simulink model "fzinfer_example"  (Simulink 6.2)
settings: Solver=ode45  StartTime=0.0  StopTime=4  FixedStep=.25  RelTol=1e-3
undefined symbols (not defined in the file): mfs, rls
libraries: simulink x1
settings Model: Creator=lbusoniu  LastModifiedBy=Administrator  ExtModeAutoUpdateStatusClock=off
settings DataIOCC: SignalLoggingName=sigsOut
settings HardwareCC: TargetUnknown=on

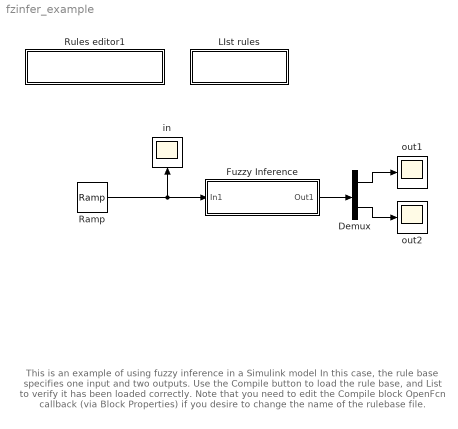
== system fzinfer_example ==
  note: This is an example of using fuzzy inference in a Simulink model
      |
      | In this case, the rule base specifies one input and two outputs.
      | Use the Compile button to load the rule base, and List to verify
      | it has been loaded correctly. Note that you need to edit the
      | Compile block OpenFcn callback (via Block Properties)
      | if you desire to change the name of the rulebase file.
  Demux : Demux  Outputs=2
  Fuzzy Inference : Subsystem  mask(Fuzzy inference block){rls=rls, mfs=mfs, def=[1 3]}
      mask prompts: rls "Rule matrix:"; mfs "Membership functions matrix:"; def "Default output:"
      mask help:
      | MIN-MAX inference with
      |  fuzzy means defuzzification
      mask Help: Fuzzy inference block can be used as a direct fuzzy controller or as a fuzzy supervisor. For details on dialog parameters see INFER.
      mask Display: disp('Fuzzy Inference')
  LIst rules : Subsystem  Orientation=down
      settings: OpenFcn=disp(rls2txt(rls, mfs, inputs, outputs, nlab, labels));
      mask Display: disp('List Fuzzy Rules')
  Ramp : simulink/Sources/Ramp  slope=1  start=0  X0=0
  Rules editor1 : Subsystem  Orientation=down
      settings: OpenFcn=eval(['[rls, mfs, inputs, outputs, nlab, labels] = txt2rls(''rulebase.rb'');']);
      mask Type: Rule-base editor
      mask Display: disp('Compile Rulebase')
  in : Scope
      settings: Orientation=up  TimeRange=4  YMin=0  YMax=4  SaveName=ScopeData2
  out1 : Scope
      settings: TimeRange=4  YMin=0  YMax=4
  out2 : Scope
      settings: TimeRange=4  YMin=0  YMax=3
  wires:
  Fuzzy Inference/1(Out1) -> Demux/1
  Demux/1 -> out1/1
  Demux/2 -> out2/1
  Ramp/1 -> Fuzzy Inference/1(In1), in/1

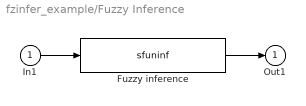
== system fzinfer_example/Fuzzy Inference ==
  In1 : Inport  Port=1  LatchInput=off
  Fuzzy inference : S-Function  FunctionName=sfuninf  Parameters=rls, mfs, def
  Out1 : Outport
  wires:
  In1/1 -> Fuzzy inference/1
  Fuzzy inference/1 -> Out1/1

== system fzinfer_example/LIst rules ==

== system fzinfer_example/Rules editor1 ==
